simulink model "lab2"  (R2019a)
settings: Solver=VariableStepAuto  StartTime=0.0  StopTime=10  RelTol=1e-3
settings Model: Creator=sumli  LastModifiedBy=sumli

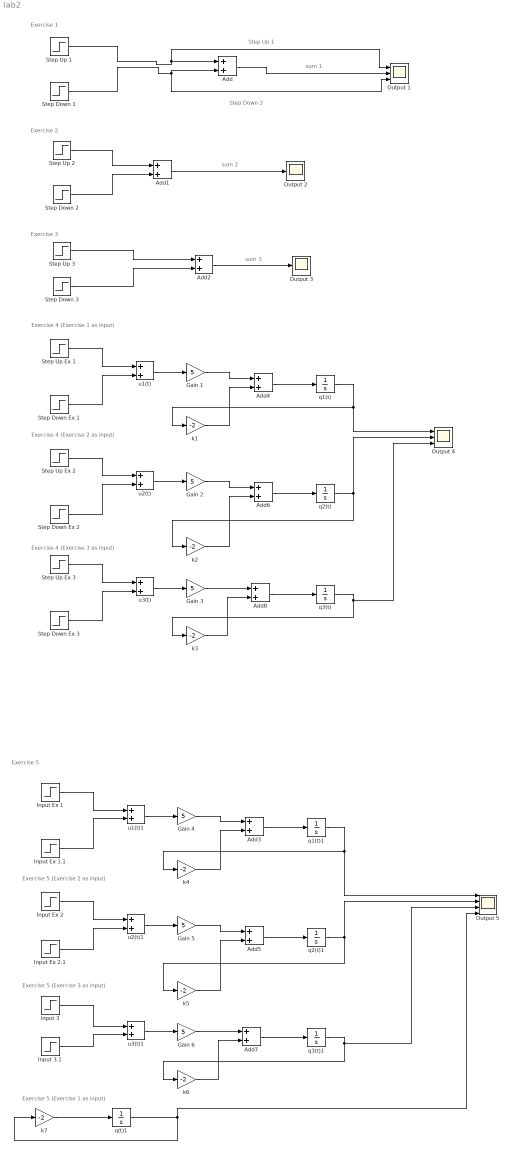
== system lab2 ==
  note: Exercise 5
  note: sum 3
  note: sum 2
  note: sum 1
  note: Step Down 2
  note: Step Up 1
  note: Exercise 4 (Exercise 1 as input)
  note: Exercise 3
  note: Exercise 2
  note: Exercise 1
  note: Exercise 4 (Exercise 2 as input)
  note: Exercise 4 (Exercise 3 as input)
  note: Exercise 5 (Exercise 2 as input)
  note: Exercise 5 (Exercise 3 as input)
  note: Exercise 5 (Exercise 1 as input)
  Add{,1..8} (9 alike) : Sum
  Gain {1..6} (6 alike) : Gain  Gain=5
  Input 3 : Step  Time=0  After=1000000  SampleTime=0
  Input 3.1 : Step  Time=0.000001  After=-1000000  SampleTime=0
  Input Ex 1 : Step  Time=0  After=0.5  SampleTime=0
  Input Ex 1.1 : Step  Time=2  After=-0.5  SampleTime=0
  Input Ex 2 : Step  Time=0  After=2  SampleTime=0
  Input Ex 2.1 : Step  Time=0.5  After=-2  SampleTime=0
  Output 1 : Scope  NumInputPorts=3
  Output 2 : Scope
  Output 3 : Scope
  Output 4 : Scope  NumInputPorts=3
  Output 5 : Scope  NumInputPorts=4
  Step Down 1 : Step  Time=2  After=-0.5  SampleTime=0
  Step Down 2 : Step  Time=0.5  After=-2  SampleTime=0
  Step Down 3 : Step  Time=0.000001  After=-1000000  SampleTime=0
  Step Down Ex 1 : Step  Time=2  After=-0.5  SampleTime=0
  Step Down Ex 2 : Step  Time=0.5  After=-2  SampleTime=0
  Step Down Ex 3 : Step  Time=0.000001  After=-1000000  SampleTime=0
  "Step Up 1 " : Step  Time=0  After=0.5  SampleTime=0
  Step Up 2 : Step  Time=0  After=2  SampleTime=0
  Step Up 3 : Step  Time=0  After=1000000  SampleTime=0
  Step Up Ex 1 : Step  Time=0  After=0.5  SampleTime=0
  Step Up Ex 2 : Step  Time=0  After=2  SampleTime=0
  Step Up Ex 3 : Step  Time=0  After=1000000  SampleTime=0
  k{1..7} (7 alike) : Gain  Gain=-2
  q(t)1 : Integrator  InitialCondition=5.5
  q1(t) : Integrator  InitialCondition=0.5
  q1(t)1 : Integrator  InitialCondition=0.5
  q2(t) : Integrator  InitialCondition=0.5
  q2(t)1 : Integrator  InitialCondition=0.5
  q3(t) : Integrator  InitialCondition=0.5
  q3(t)1 : Integrator  InitialCondition=0.5
  u1(t) : Sum
  u1(t)1 : Sum
  u2(t) : Sum
  u2(t)1 : Sum
  u3(t) : Sum
  u3(t)1 : Sum
  wires:
  "Step Up 1 "/1 -> Output 1/1, Add/1
  Step Down 1/1 -> Output 1/3, Add/2
  Step Up 2/1 -> Add1/1
  Step Down 2/1 -> Add1/2
  Add1/1 -> Output 2/1
  Step Up 3/1 -> Add2/1
  Step Down 3/1 -> Add2/2
  Add2/1 -> Output 3/1
  Step Up Ex 1/1 -> u1(t)/1
  Step Down Ex 1/1 -> u1(t)/2
  Add/1 -> Output 1/2
  u1(t)/1 -> Gain 1/1
  Gain 1/1 -> Add4/1
  k1/1 -> Add4/2
  Add4/1 -> q1(t)/1
  q1(t)/1 -> Output 4/1, k1/1
  Step Up Ex 2/1 -> u2(t)/1
  Step Down Ex 2/1 -> u2(t)/2
  u2(t)/1 -> Gain 2/1
  q2(t)/1 -> Output 4/2, k2/1
  Gain 2/1 -> Add6/1
  Add6/1 -> q2(t)/1
  k2/1 -> Add6/2
  q3(t)/1 -> Output 4/3, k3/1
  Step Up Ex 3/1 -> u3(t)/1
  k3/1 -> Add8/2
  Step Down Ex 3/1 -> u3(t)/2
  Gain 3/1 -> Add8/1
  u3(t)/1 -> Gain 3/1
  Add8/1 -> q3(t)/1
  Input Ex 1.1/1 -> u1(t)1/2
  Add7/1 -> q3(t)1/1
  q2(t)1/1 -> Output 5/2, k5/1
  Input Ex 2/1 -> u2(t)1/1
  Gain 5/1 -> Add5/1
  Add3/1 -> q1(t)1/1
  Gain 4/1 -> Add3/1
  k5/1 -> Add5/2
  k4/1 -> Add3/2
  u2(t)1/1 -> Gain 5/1
  Input 3/1 -> u3(t)1/1
  Input Ex 1/1 -> u1(t)1/1
  u1(t)1/1 -> Gain 4/1
  Input Ex 2.1/1 -> u2(t)1/2
  Add5/1 -> q2(t)1/1
  u3(t)1/1 -> Gain 6/1
  Gain 6/1 -> Add7/1
  q1(t)1/1 -> Output 5/1, k4/1
  Input 3.1/1 -> u3(t)1/2
  q3(t)1/1 -> Output 5/3, k6/1
  k6/1 -> Add7/2
  k7/1 -> q(t)1/1
  q(t)1/1 -> Output 5/4, k7/1
